simulink model "cruise_control"  (R2017b)
settings: Solver=VariableStepAuto  StartTime=0.0  StopTime=10.0  RelTol=1e-3
PreLoadFcn:
  | load('cruise_control.mat')
values from neighbouring files (symbols this model uses):
  Ki = 1    [alfa147gta.mat]    (also in cruise_control.mat; cruise_control_sim.mat = 0)
  Kp = 1    [alfa147gta.mat]    (also in cruise_control.mat; cruise_control_sim.mat = 0.4)
settings Model: Creator=Michele  LastModifiedBy=Michele

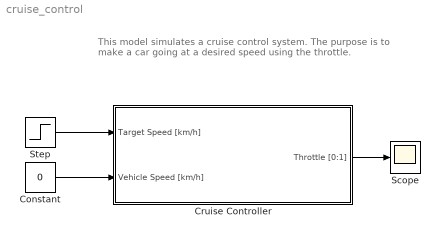
== system cruise_control ==
  note: This model simulates a cruise control system. The purpose is to make a car going at a desired speed using the throttle.
  Constant : Constant  Value=0
  Cruise Controller : Subsystem
  Scope : Scope
  Step : Step  After=.1  SampleTime=0
  wires:
  Step/1 -> Cruise Controller/1(Target Speed [km/h])
  Constant/1 -> Cruise Controller/2("Vehicle Speed [km/h] ")
  Cruise Controller/1("Throttle [0:1] ") -> Scope/1

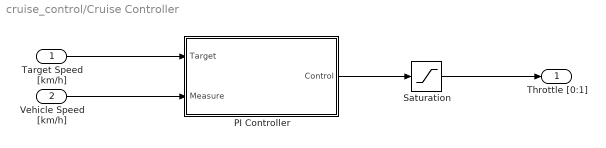
== system cruise_control/Cruise Controller ==
  Target Speed [km/h] : Inport
  "Vehicle Speed [km/h] " : Inport  Port=2
  PI Controller : Subsystem
  Saturation : Saturate  UpperLimit=1  LowerLimit=0
  "Throttle [0:1] " : Outport
  wires:
  "Vehicle Speed [km/h] "/1 -> PI Controller/2(Measure)
  PI Controller/1(Control) -> Saturation/1
  Target Speed [km/h]/1 -> PI Controller/1(Target)
  Saturation/1 -> "Throttle [0:1] "/1

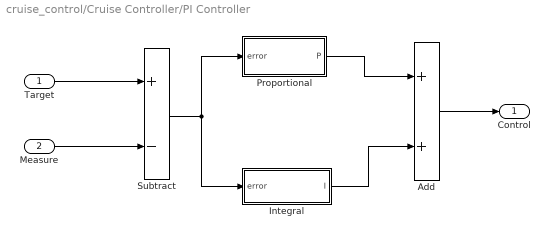
== system cruise_control/Cruise Controller/PI Controller ==
  Target : Inport
  Measure : Inport  Port=2
  Add : Sum
  Integral : Subsystem
  Proportional : Subsystem
  Subtract : Sum  Inputs=+-
  Control : Outport
  wires:
  Integral/1(I) -> Add/2
  Add/1 -> Control/1
  Proportional/1(P) -> Add/1
  Target/1 -> Subtract/1
  Measure/1 -> Subtract/2
  Subtract/1 -> Proportional/1(error), Integral/1(error)

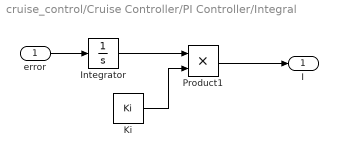
== system cruise_control/Cruise Controller/PI Controller/Integral ==
  error : Inport
  Integrator : Integrator
  Ki : Constant  Value=Ki
  Product1 : Product
  I : Outport
  wires:
  error/1 -> Integrator/1
  Ki/1 -> Product1/2
  Integrator/1 -> Product1/1
  Product1/1 -> I/1

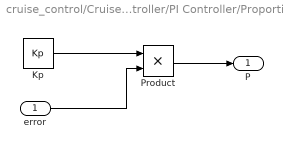
== system cruise_control/Cruise Controller/PI Controller/Proportional ==
  error : Inport
  Kp : Constant  Value=Kp
  Product : Product
  P : Outport
  wires:
  Kp/1 -> Product/1
  error/1 -> Product/2
  Product/1 -> P/1
